simulink model "testt"  (R2018b)
settings: Solver=VariableStepAuto  StartTime=0.0  StopTime=10.0  RelTol=1e-3
settings Model: Creator=BMT Group  LastModifiedBy=BMT Group

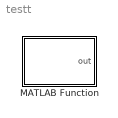
== system testt ==
  MATLAB Function : MATLAB Function  TreatAsAtomicUnit=on

== matlab function testt/MATLAB Function ==
  data: out output
function out = fcn()
setting_simulink

out =0
